simulink model "lab4_monocontur"  (R2023b)
settings: Solver=ode45  StartTime=0.0  StopTime=150  RelTol=1e-3
settings Model: Creator=Daniela  LastModifiedBy=Daniela

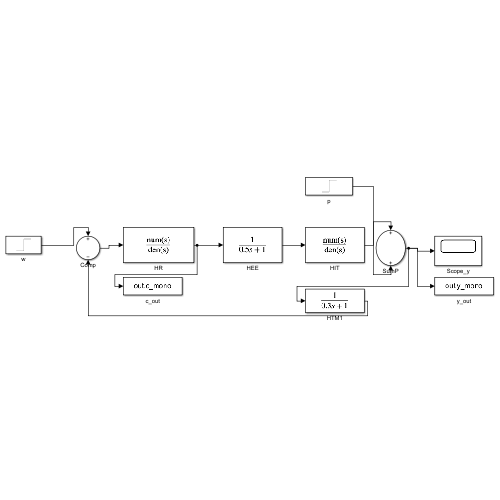
[thumbnail: Simulink's stored preview of the top-level diagram]
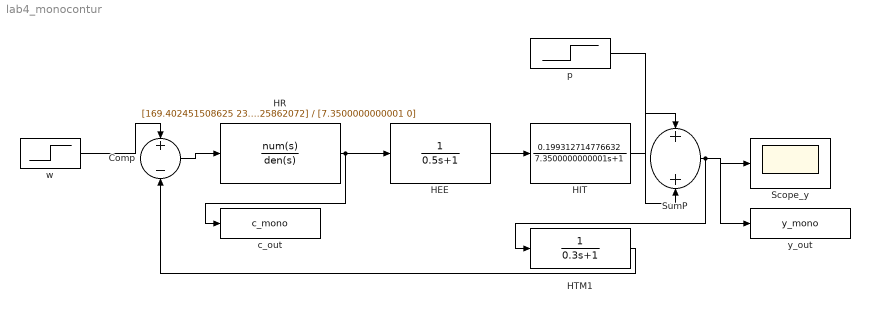
== system lab4_monocontur ==
  Comp : Sum  Inputs=+-
  HEE : TransferFcn  Numerator=1  Denominator=[0.5 1]
  HIT : TransferFcn  Numerator=0.199312714776632  Denominator=[7.3500000000001 1]
  HR : TransferFcn  Numerator=[169.402451508625 23.0479525862072]  Denominator=[7.3500000000001 0]
  HTM1 : TransferFcn  Numerator=1  Denominator=[0.3 1]
  Scope_y : Scope
  SumP : Sum
  c_out : ToWorkspace  VariableName=c_mono  SampleTime=-1
  p : Step  Time=50  SampleTime=0
  w : Step  Time=0  SampleTime=0
  y_out : ToWorkspace  VariableName=y_mono  SampleTime=-1
  wires:
  w/1 -> Comp/1
  Comp/1 -> HR/1
  HR/1 -> HEE/1, c_out/1
  HEE/1 -> HIT/1
  HIT/1 -> SumP/1
  p/1 -> SumP/2
  SumP/1 -> Scope_y/1, y_out/1, HTM1/1
  HTM1/1 -> Comp/2
